simulink model "Kite"  (R2017b)
settings: Solver=VariableStepAuto  StartTime=0.0  StopTime=60  RelTol=1e-3  EnableMultiTasking=on
values from neighbouring files (symbols this model uses):
  A = 0.28    [init.m]    (also in main.m)
  beta0 = beta_star+betinho*pi/180    (= 0.436332312999)    [init.m]    (also in main.m)
  beta_star = 40*pi/180    (= 0.698131700798)    [init.m]    (also in main.m)
  beta_total = [y1 y2 y3 y4]    [init.m]    (also in main.m)
  dbeta0 = 0*pi/180    (= 0)    [init.m]    (also in main.m)
  delta_phi = 20*pi/180    (= 0.349065850399)    [init.m]    (also in main.m)
  dphi0 = -0.1*pi/180    (= -0.00174532925199)    [init.m]    (also in main.m)
  dr0 = 0    [init.m]    (also in main.m)
  g = 9.8    [init.m]    (also in main.m)
  imax = size    [init.m]    (also in main.m)
  L0 = L_0*pi/180    [init.m]    (also in main.m)
  m = 0.7    [init.m]    (also in main.m)
  phi0 = phi_star+phizinho*pi/180    (= 0.523598775598)    [init.m]    (also in main.m)
  phi_total = [x1 x2 x3 x4]    [init.m]    (also in main.m)
  r0 = rmin    (= 50)    [init.m]    (also in main.m)
  rmax = 275    [init.m]    (also in main.m = 250)
  rmin = 50    [init.m]    (also in main.m)
  Ro = 1.2    [init.m]    (also in main.m)
  vw = 10    [init.m]    (also in main.m)
settings Model: Creator=Gonçalo  LastModifiedBy=Conrado
settings SolverCC: MaxConsecutiveMinStep=10
settings OptimizationCC: LifeSpan=inf
settings DebuggingCC: SFUnexpectedBacktrackingDiag=warning  SFNoUnconditionalDefaultTransitionDiag=warning  SFExecutionAtInitializationDiag=none
settings CodeAppCC: StateflowObjectComments=on
settings GRTTargetCC: TargetLangStandard=C89/C90 (ANSI)
settings ConfigComp: CovMetricSettings=dw  CovSaveCumulativeToWorkspaceVar=on  CovSaveSingleToWorkspaceVar=on  CovExternalEMLEnable=off

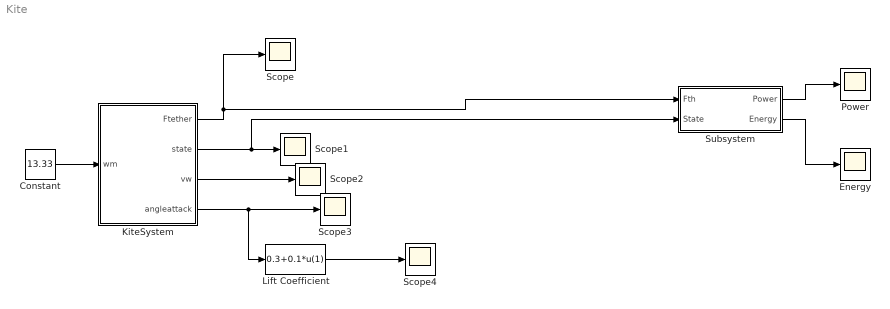
== system Kite ==
  Constant : Constant  Value=13.33
  "Energy " : Scope
  KiteSystem : Subsystem
  Lift Coefficient : Fcn  Expr=0.3+0.1*u(1)
  Power : Scope
  Scope{,1..4} (5 alike) : Scope
  Subsystem : Subsystem
  wires:
  Constant/1 -> KiteSystem/1(wm)
  KiteSystem/3("vw ") -> Scope2/1
  KiteSystem/4(angleattack) -> Lift Coefficient/1, Scope3/1
  Lift Coefficient/1 -> Scope4/1
  Subsystem/2("Energy ") -> "Energy "/1
  KiteSystem/2(state) -> Subsystem/2(State), Scope1/1
  Subsystem/1("Power ") -> Power/1
  KiteSystem/1(Ftether) -> Subsystem/1("Fth "), Scope/1

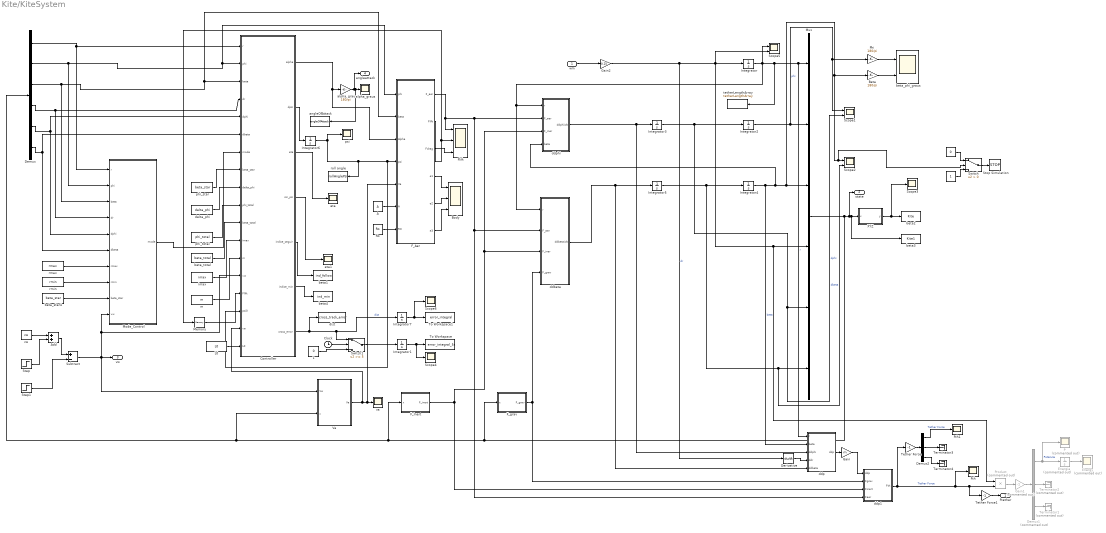
== system Kite/KiteSystem ==
  wm : Inport
  " " : Constant  Value=0
  " " : Constant
  " 1" : Constant  Value=0
  A : Constant  Value=A
  Add : Sum
  Beta : Gain  Gain=180/pi
  Body : Scope  NumInputPorts=3
  Clock : Clock
  Controller : MATLAB Function  TreatAsAtomicUnit=on
  Demux : Demux  Outputs=6
  Demux1 : Demux  Commented=on  Outputs=3
  Demux2 : Demux  Outputs=3
  Derivative : Derivative
  Energia : Integrator  Commented=on
  Energy : Scope  Commented=on
  F_Aer : Subsystem
  F_Inert : Subsystem
  F_grav : Subsystem
  Flift : Scope  NumInputPorts=3
  Fth : Scope
  Fth1 : Scope
  Gain : Gain  Gain=m
  Gain1 : Gain  Commented=on  Gain=-1
  Gain2 : Gain  Gain=0.25
  Integrator : Integrator  InitialCondition=r0
  Integrator1 : Integrator
  Integrator2 : Integrator  InitialCondition=phi0
  Integrator3 : Integrator  InitialCondition=dphi0
  Integrator4 : Integrator  InitialCondition=beta0
  Integrator5 : Integrator  InitialCondition=dbeta0
  Integrator6 : Integrator  InitialCondition=dr0
  Integrator7 : Integrator
  L0 : Constant  Value=L0
  Memory : Memory  InitialCondition=300
  Mode_Control : MATLAB Function  TreatAsAtomicUnit=on
  Mux : Mux  Inputs=6
  P : Scope  Commented=on
  Phi : Gain  Gain=180/pi
  Product : Product  Commented=on
  Ro : Constant  Value=Ro
  Scope1 : Scope  NumInputPorts=2
  Scope2 : Scope  NumInputPorts=2
  Scope3 : Scope
  Scope4 : Scope
  Scope5 : Scope  NumInputPorts=2
  Scope6 : Scope
  Step : Step  Time=25  After=0  SampleTime=0
  Step1 : Step  Time=27  After=0  SampleTime=0
  Stop Simulation : Stop
  Subtract : Sum  Inputs=+-
  Switch : Switch  Criteria=u2 > Threshold
  Switch1 : Switch  Threshold=5
  Terminator1 : Terminator  Commented=on
  Terminator2 : Terminator  Commented=on
  Terminator3 : Terminator
  Terminator4 : Terminator
  Tether Force : Gain  Gain=-1
  Tether Force1 : Gain  Gain=-1
  To Workspace : ToWorkspace  VariableName=error_integral_5s  SampleTime=-1
      settings: Save2DSignal=2-D array (concatenate along first dimension)
  To Workspace1 : ToWorkspace  VariableName=error_integral  SampleTime=-1
      settings: Save2DSignal=2-D array (concatenate along first dimension)
  Va : Subsystem
  XYZ : MATLAB Function  TreatAsAtomicUnit=on
  alpha_grau : Gain  Gain=180/pi
  alpha_graus : Scope
  angleOfAttack : ToWorkspace  VariableName=angleOfAttack  SampleTime=-1
      settings: Save2DSignal=2-D array (concatenate along first dimension)
  beta1 : ToWorkspace  VariableName=ind_follow  SampleTime=-1
      settings: Save2DSignal=2-D array (concatenate along first dimension)
  beta2 : ToWorkspace  VariableName=Kite  SampleTime=-1
      settings: Save2DSignal=2-D array (concatenate along first dimension)
  beta3 : ToWorkspace  VariableName=Kite1  SampleTime=-1
      settings: Save2DSignal=2-D array (concatenate along first dimension)
  beta4 : ToWorkspace  VariableName=ind_min  SampleTime=-1
      settings: Save2DSignal=2-D array (concatenate along first dimension)
  "beta_phi_graus " : Scope  NumInputPorts=2
  beta_star4 : Constant  Value=beta_star
  beta_total : Constant  Value=beta_total
  ddbeta : Subsystem
  ddp : Subsystem
  ddp1 : Subsystem
  ddphi : Subsystem
  delta_phi : Constant  Value=delta_phi
  dist : ToWorkspace  VariableName=cross_track_error  SampleTime=-1
      settings: Save2DSignal=2-D array (concatenate along first dimension)
  eta : Scope
  eta1 : Scope
  imax : Constant  Value=imax
  m : Constant  Value=m
  phi_star : Constant  Value=beta_star
  phi_total : Constant  Value=phi_total
  psi : Scope
  "rmax " : Constant  Value=rmax
  "rmin " : Constant  Value=rmin
  roll angle : ToWorkspace  VariableName=rollAnglePsi  SampleTime=-1
      settings: Save2DSignal=2-D array (concatenate along first dimension)
  tetherLengthArray : ToWorkspace  VariableName=tetherLengthArray  SampleTime=-1
      settings: Save2DSignal=2-D array (concatenate along first dimension)
  va : Scope
  vw : Constant  Value=vw
  Ftether : Outport
  state : Outport  Port=2
  "vw " : Outport  Port=3
  angleattack : Outport  Port=4
  wires:
  Integrator2/1 -> Scope1/1, Phi/1, Mux/2  "phi"
  Mode_Control/1(mode) -> Controller/7(mode)
  Integrator/1 -> Scope5/1, tetherLengthArray/1, ddp/1("r "), Mux/1, ddbeta/1(r), ddphi/1(r)  "r"
  beta_total/1 -> Controller/11(beta_total)
  imax/1 -> Controller/12(imax)
  Phi/1 -> "beta_phi_graus "/1
  Demux/1 -> Mode_Control/1(r), Controller/1(r)
  phi_star/1 -> Controller/8(beta_star)
  Subtract/1 -> "vw "/1, Controller/14(vw), Mode_Control/10(vw), Va/1("Vw ")
  Beta/1 -> "beta_phi_graus "/2
  Product/1 -> Gain1/1
  Demux/4 -> Mode_Control/4(dr), Controller/4(dr)
  phi_total/1 -> Controller/10(phi_total)
  Demux/2 -> Mode_Control/2(phi), Controller/2(phi), F_Aer/1("phi ")
  Demux1/3 -> Terminator1/1
  XYZ/1(y) -> Scope3/1, beta2/1
  A/1 -> F_Aer/6(A)
  Gain2/1 -> Derivative/1, Scope5/2, Product/1, Mux/4, Integrator/1  "dr"
  Mux/1 -> F_Inert/1("x "), Va/2(x), Demux/1, F_grav/1("x "), state/1, beta3/1, XYZ/1(x)
  Controller/2(dpsi) -> Integrator6/1
  ddp/1("ddp ") -> Gain/1
  ddbeta/1("ddbeta/dt ") -> Integrator5/1, ddp/5(ddbeta)
  Demux/3 -> Mode_Control/3(beta), F_Aer/2(beta), Controller/3(beta)
  F_Inert/1("F_inert ") -> ddphi/3(F_iner), ddbeta/3(F_iner), ddp1/3(Finert)
  Integrator4/1 -> ddp/2(beta), ddphi/4(beta), Switch/2, Scope2/1, Beta/1, Mux/3  "beta"
  ddphi/1("ddphi/dt ") -> ddp/3("ddphi "), Integrator3/1
  Integrator3/1 -> Integrator2/1, Scope1/2, Mux/5  "dphi"
  Integrator5/1 -> Integrator4/1, Scope2/2, Mux/6  "dbeta"
  Demux/5 -> Mode_Control/5(dphi), Controller/5(dphi)
  F_Aer/2(Flift) -> Flift/2, Memory/1
  Demux2/3 -> Terminator4/1
  F_Aer/3(Fdrag) -> Flift/3
  delta_phi/1 -> Controller/9(delta_phi)
  F_Aer/1("F_aer ") -> ddp1/4("Faer "), ddbeta/2(F_aer), ddphi/2(F_aer), Flift/1
  Demux/6 -> Mode_Control/6(dbeta), Controller/6(dbeta)
  m/1 -> Controller/13(m)
  Step/1 -> Add/2
  Ro/1 -> F_Aer/7(R0)
  vw/1 -> Add/1
  Controller/1(alpha) -> alpha_grau/1, F_Aer/3(Alpha)
  Gain1/1 -> Demux1/1
  Demux1/2 -> Terminator2/1
  "rmin "/1 -> Mode_Control/8(rmin)
  Demux1/1 -> P/1, Energia/1  "Potência"
  F_Aer/6(e3) -> Body/3
  Tether Force/1 -> Demux2/1
  Integrator6/1 -> roll angle/1, Controller/16(psi0), F_Aer/4(psi), psi/1
  "rmax "/1 -> Mode_Control/7(rmax)
  F_Aer/4(e1) -> Body/1
  Va/1("Va ") -> Controller/17(va), va/1, F_Aer/5(Va)
  F_Aer/5(e2) -> Body/2
  Add/1 -> Subtract/1
  Memory/1 -> Controller/15(Flift)
  Gain/1 -> ddp1/1(ddp)
  F_grav/1("F_grav ") -> ddbeta/4(F_grav), ddp1/2(Fgrav)
  " "/1 -> Switch/1
  beta_star4/1 -> Mode_Control/9(beta_star)
  Demux2/1 -> Fth1/1  "Tether Force"
  Energia/1 -> Energy/1
  " "/1 -> Switch/3
  Demux2/2 -> Terminator3/1
  Step1/1 -> Subtract/2
  Switch/1 -> Stop Simulation/1
  wm/1 -> Gain2/1
  Derivative/1 -> ddp/4(ddr)
  alpha_grau/1 -> angleattack/1, angleOfAttack/1, alpha_graus/1
  ddp1/1("Fth ") -> Tether Force1/1, Product/2, Fth/1, Tether Force/1  "Tether Force"
  Tether Force1/1 -> Ftether/1
  Controller/4(sin_psi) -> eta1/1
  Controller/3(eta) -> eta/1
  Controller/5(indice_seguir) -> beta1/1
  Controller/6(indice_min) -> beta4/1
  L0/1 -> Controller/18(L0)
  Controller/7(cross_error) -> Switch1/1, Integrator7/1, dist/1  "dist"
  Integrator1/1 -> To Workspace/1, Scope4/1
  Switch1/1 -> Integrator1/1
  Clock/1 -> Switch1/2
  Integrator7/1 -> Scope6/1, To Workspace1/1
  " 1"/1 -> Switch1/3

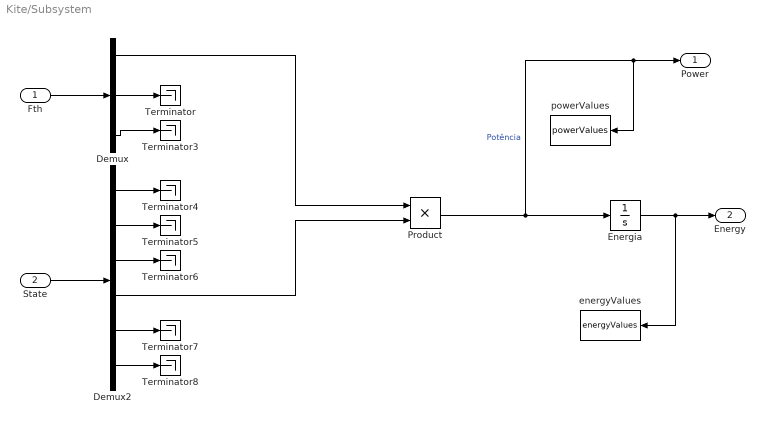
== system Kite/Subsystem ==
  "Fth " : Inport
  State : Inport  Port=2
  Demux : Demux  Outputs=3
  Demux2 : Demux  Outputs=6
  Energia : Integrator
  Product : Product
  Terminator{,3..8} (7 alike) : Terminator
  energyValues : ToWorkspace  VariableName=energyValues  SampleTime=-1
      settings: Save2DSignal=2-D array (concatenate along first dimension)
  powerValues : ToWorkspace  VariableName=powerValues  SampleTime=-1
      settings: Save2DSignal=2-D array (concatenate along first dimension)
  "Power " : Outport
  "Energy " : Outport  Port=2
  wires:
  Product/1 -> Energia/1, powerValues/1, "Power "/1  "Potência"
  Energia/1 -> energyValues/1, "Energy "/1
  "Fth "/1 -> Demux/1
  State/1 -> Demux2/1
  Demux/2 -> Terminator/1
  Demux/3 -> Terminator3/1
  Demux2/1 -> Terminator4/1
  Demux2/2 -> Terminator5/1
  Demux2/3 -> Terminator6/1
  Demux2/5 -> Terminator7/1
  Demux2/6 -> Terminator8/1
  Demux2/4 -> Product/2
  Demux/1 -> Product/1

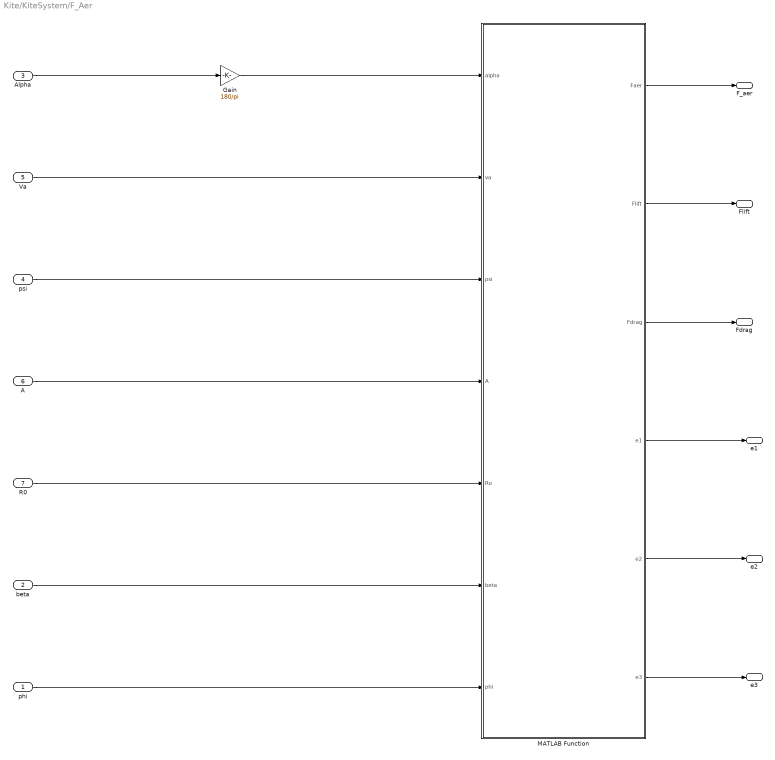
== system Kite/KiteSystem/F_Aer ==
  "phi " : Inport
  beta : Inport  Port=2
  Alpha : Inport  Port=3
  psi : Inport  Port=4
  Va : Inport  Port=5
  A : Inport  Port=6
  R0 : Inport  Port=7
  Gain : Gain  Gain=180/pi
  MATLAB Function : MATLAB Function  TreatAsAtomicUnit=on
  "F_aer " : Outport
  Flift : Outport  Port=2
  Fdrag : Outport  Port=3
  e1 : Outport  Port=4
  e2 : Outport  Port=5
  e3 : Outport  Port=6
  wires:
  Alpha/1 -> Gain/1
  Va/1 -> MATLAB Function/2(va)
  psi/1 -> MATLAB Function/3(psi)
  A/1 -> MATLAB Function/4(A)
  R0/1 -> MATLAB Function/5(Ro)
  MATLAB Function/1(Faer) -> "F_aer "/1
  beta/1 -> MATLAB Function/6(beta)
  "phi "/1 -> MATLAB Function/7(phi)
  Gain/1 -> MATLAB Function/1(alpha)
  MATLAB Function/2(Flift) -> Flift/1
  MATLAB Function/3(Fdrag) -> Fdrag/1
  MATLAB Function/4(e1) -> e1/1
  MATLAB Function/5(e2) -> e2/1
  MATLAB Function/6(e3) -> e3/1

== system Kite/KiteSystem/F_Inert ==
  "x " : Inport
  Add : Sum
  Fcent : Subsystem
  Fcor : Subsystem
  "F_inert " : Outport
  wires:
  Add/1 -> "F_inert "/1
  "x "/1 -> Fcent/1(x), Fcor/1(x)
  Fcent/1(Fcent) -> Add/1
  Fcor/1(Fcor) -> Add/2

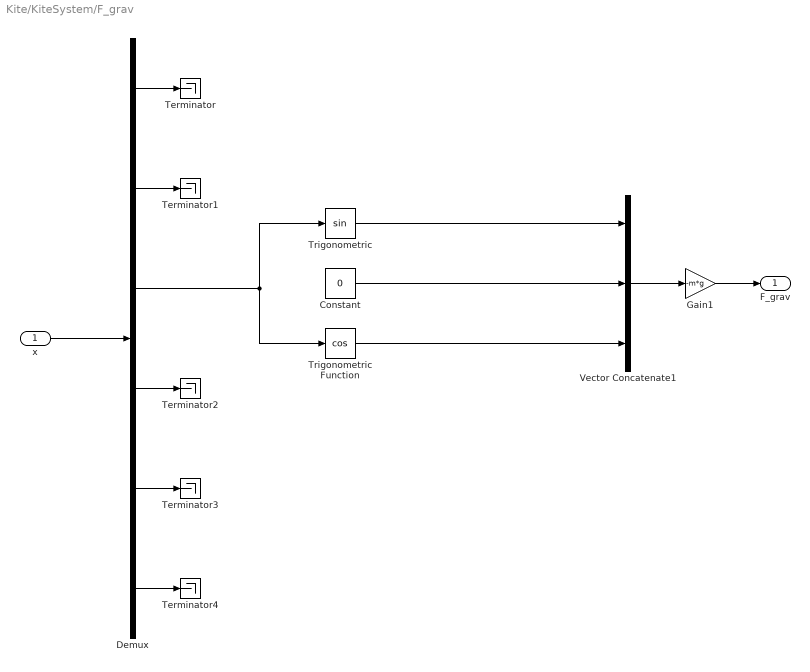
== system Kite/KiteSystem/F_grav ==
  "x " : Inport
  Constant : Constant  Value=0
  Demux : Demux  Outputs=6
  Gain1 : Gain  Gain=-m*g
  Terminator{,1..4} (5 alike) : Terminator
  Trigonometric : Trigonometry
  Trigonometric Function : Trigonometry  Operator=cos
  Vector Concatenate1 : Concatenate  NumInputs=3  Mode=Multidimensional array
  "F_grav " : Outport
  wires:
  Vector Concatenate1/1 -> Gain1/1
  Gain1/1 -> "F_grav "/1
  Trigonometric/1 -> Vector Concatenate1/1
  Demux/1 -> Terminator/1
  Demux/3 -> Trigonometric Function/1, Trigonometric/1
  Demux/4 -> Terminator2/1
  "x "/1 -> Demux/1
  Demux/2 -> Terminator1/1
  Demux/5 -> Terminator3/1
  Demux/6 -> Terminator4/1
  Trigonometric Function/1 -> Vector Concatenate1/3
  Constant/1 -> Vector Concatenate1/2

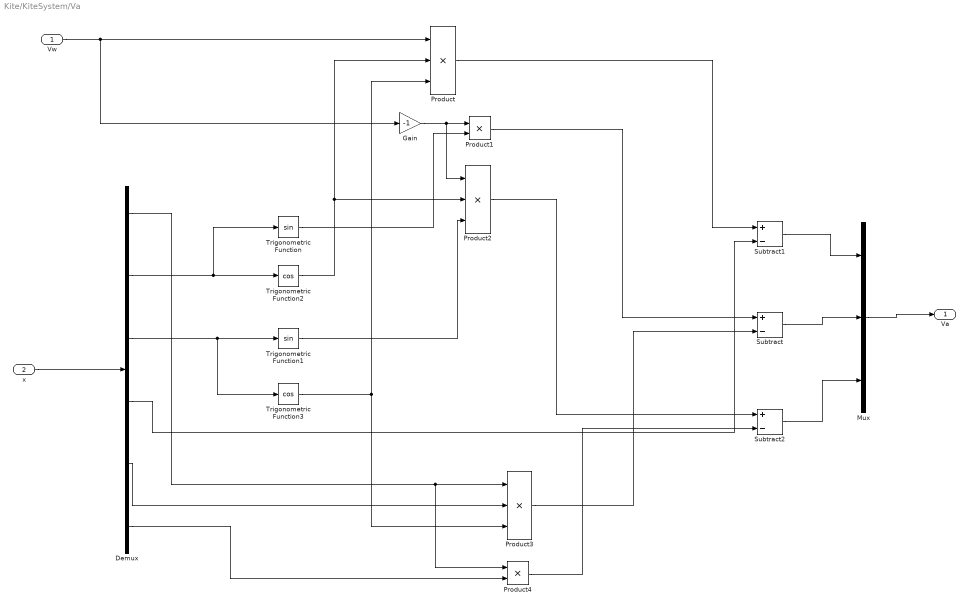
== system Kite/KiteSystem/Va ==
  "Vw " : Inport
  x : Inport  Port=2
  Demux : Demux  Outputs=6
  Gain : Gain  Gain=-1
  Mux : Mux  Inputs=3
  Product : Product  Inputs=3
  Product1 : Product
  Product2 : Product  Inputs=3
  Product3 : Product  Inputs=3
  Product4 : Product
  Subtract : Sum  Inputs=+-
  Subtract1 : Sum  Inputs=+-
  Subtract2 : Sum  Inputs=+-
  Trigonometric Function : Trigonometry
  Trigonometric Function1 : Trigonometry
  Trigonometric Function2 : Trigonometry  Operator=cos
  Trigonometric Function3 : Trigonometry  Operator=cos
  "Va " : Outport
  wires:
  x/1 -> Demux/1
  Demux/2 -> Trigonometric Function2/1, Trigonometric Function/1
  Demux/3 -> Trigonometric Function3/1, Trigonometric Function1/1
  "Vw "/1 -> Gain/1, Product/1
  Trigonometric Function2/1 -> Product2/2, Product/2
  Trigonometric Function3/1 -> Product3/3, Product/3
  Product1/1 -> Subtract/1
  Product/1 -> Subtract1/1
  Gain/1 -> Product2/1, Product1/1
  Product3/1 -> Subtract/2
  Demux/4 -> Subtract1/2
  Demux/1 -> Product3/1, Product4/1
  Product4/1 -> Subtract2/2
  Trigonometric Function/1 -> Product1/2
  Trigonometric Function1/1 -> Product2/3
  Demux/5 -> Product3/2
  Demux/6 -> Product4/2
  Product2/1 -> Subtract2/1
  Subtract1/1 -> Mux/1
  Mux/1 -> "Va "/1
  Subtract/1 -> Mux/2
  Subtract2/1 -> Mux/3

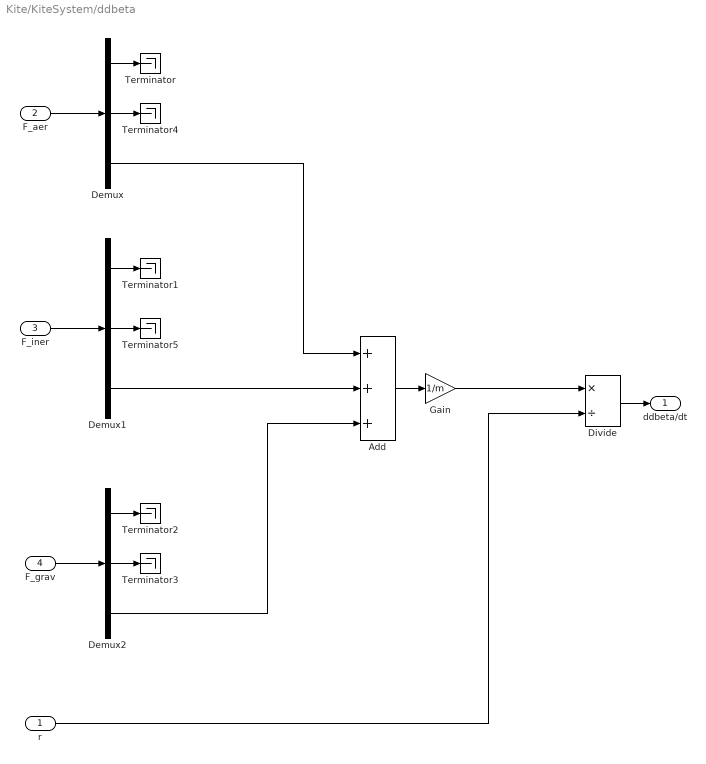
== system Kite/KiteSystem/ddbeta ==
  r : Inport
  F_aer : Inport  Port=2
  F_iner : Inport  Port=3
  F_grav : Inport  Port=4
  Add : Sum  Inputs=+++
  Demux : Demux  Outputs=3
  Demux1 : Demux  Outputs=3
  Demux2 : Demux  Outputs=3
  Divide : Product  Inputs=*/
  Gain : Gain  Gain=1/m
  Terminator{,1..5} (6 alike) : Terminator
  "ddbeta/dt " : Outport
  wires:
  Gain/1 -> Divide/1
  Add/1 -> Gain/1
  F_aer/1 -> Demux/1
  Demux/1 -> Terminator/1
  F_iner/1 -> Demux1/1
  Demux1/1 -> Terminator1/1
  Divide/1 -> "ddbeta/dt "/1
  r/1 -> Divide/2
  F_grav/1 -> Demux2/1
  Demux2/1 -> Terminator2/1
  Demux2/3 -> Add/3
  Demux2/2 -> Terminator3/1
  Demux/2 -> Terminator4/1
  Demux/3 -> Add/1
  Demux1/3 -> Add/2
  Demux1/2 -> Terminator5/1

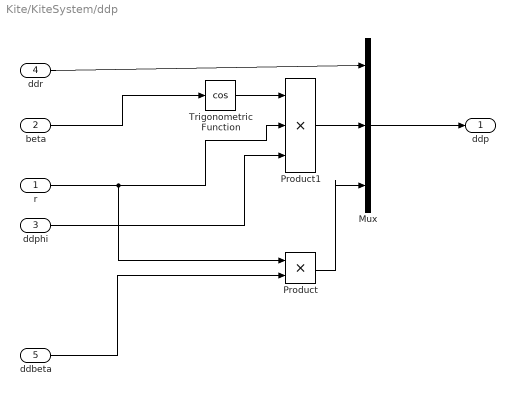
== system Kite/KiteSystem/ddp ==
  "r " : Inport
  beta : Inport  Port=2
  "ddphi " : Inport  Port=3
  ddr : Inport  Port=4
  ddbeta : Inport  Port=5
  Mux : Mux  Inputs=3
  Product : Product
  Product1 : Product  Inputs=3
  Trigonometric Function : Trigonometry  Operator=cos
  "ddp " : Outport
  wires:
  Mux/1 -> "ddp "/1
  ddr/1 -> Mux/1
  ddbeta/1 -> Product/2
  Product/1 -> Mux/3
  "r "/1 -> Product1/2, Product/1
  Product1/1 -> Mux/2
  Trigonometric Function/1 -> Product1/1
  beta/1 -> Trigonometric Function/1
  "ddphi "/1 -> Product1/3

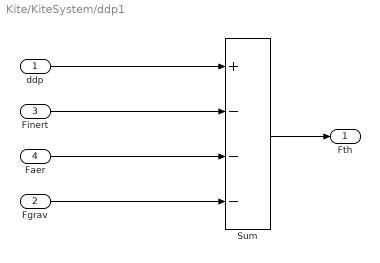
== system Kite/KiteSystem/ddp1 ==
  ddp : Inport
  Fgrav : Inport  Port=2
  Finert : Inport  Port=3
  "Faer " : Inport  Port=4
  Sum : Sum  Inputs=+---
  "Fth " : Outport
  wires:
  ddp/1 -> Sum/1
  Finert/1 -> Sum/2
  "Faer "/1 -> Sum/3
  Sum/1 -> "Fth "/1
  Fgrav/1 -> Sum/4

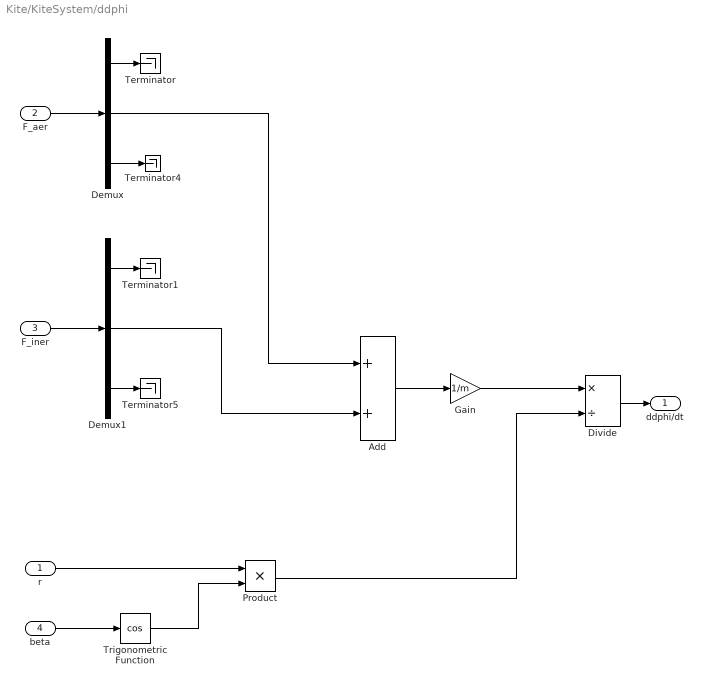
== system Kite/KiteSystem/ddphi ==
  r : Inport
  F_aer : Inport  Port=2
  F_iner : Inport  Port=3
  beta : Inport  Port=4
  Add : Sum
  Demux : Demux  Outputs=3
  Demux1 : Demux  Outputs=3
  Divide : Product  Inputs=*/
  Gain : Gain  Gain=1/m
  Product : Product
  Terminator{,1,4..5} (4 alike) : Terminator
  Trigonometric Function : Trigonometry  Operator=cos
  "ddphi/dt " : Outport
  wires:
  Gain/1 -> Divide/1
  Add/1 -> Gain/1
  F_aer/1 -> Demux/1
  Demux/1 -> Terminator/1
  F_iner/1 -> Demux1/1
  Demux1/1 -> Terminator1/1
  Divide/1 -> "ddphi/dt "/1
  Demux/3 -> Terminator4/1
  Demux1/3 -> Terminator5/1
  Demux/2 -> Add/1
  Demux1/2 -> Add/2
  beta/1 -> Trigonometric Function/1
  r/1 -> Product/1
  Trigonometric Function/1 -> Product/2
  Product/1 -> Divide/2

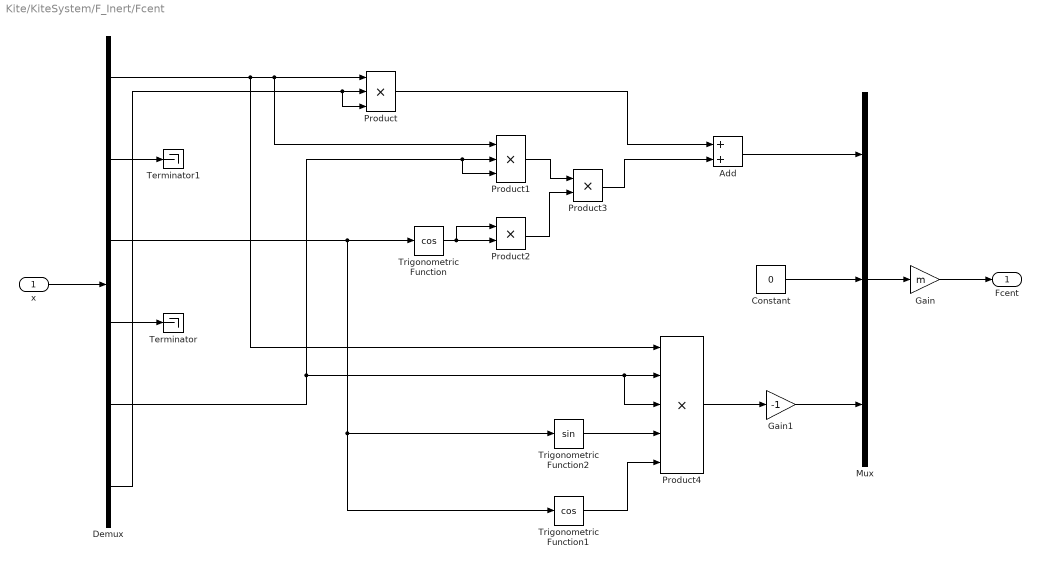
== system Kite/KiteSystem/F_Inert/Fcent ==
  x : Inport
  Add : Sum
  Constant : Constant  Value=0
  Demux : Demux  Outputs=6
  Gain : Gain  Gain=m
  Gain1 : Gain  Gain=-1
  Mux : Mux  Inputs=3
  Product : Product  Inputs=3
  Product1 : Product  Inputs=3
  Product2 : Product
  Product3 : Product
  Product4 : Product  Inputs=5
  Terminator : Terminator
  Terminator1 : Terminator
  Trigonometric Function : Trigonometry  Operator=cos
  Trigonometric Function1 : Trigonometry  Operator=cos
  Trigonometric Function2 : Trigonometry
  Fcent : Outport
  wires:
  x/1 -> Demux/1
  Gain/1 -> Fcent/1
  Mux/1 -> Gain/1
  Demux/1 -> Product4/1, Product1/1, Product/1
  Demux/3 -> Trigonometric Function1/1, Trigonometric Function2/1, Trigonometric Function/1
  Trigonometric Function/1 -> Product2/1, Product2/2
  Product1/1 -> Product3/1
  Product2/1 -> Product3/2
  Product3/1 -> Add/2
  Product/1 -> Add/1
  Add/1 -> Mux/1
  Constant/1 -> Mux/2
  Gain1/1 -> Mux/3
  Product4/1 -> Gain1/1
  Trigonometric Function2/1 -> Product4/4
  Trigonometric Function1/1 -> Product4/5
  Demux/4 -> Terminator/1
  Demux/5 -> Product4/3, Product4/2, Product1/3, Product1/2
  Demux/6 -> Product/3, Product/2
  Demux/2 -> Terminator1/1

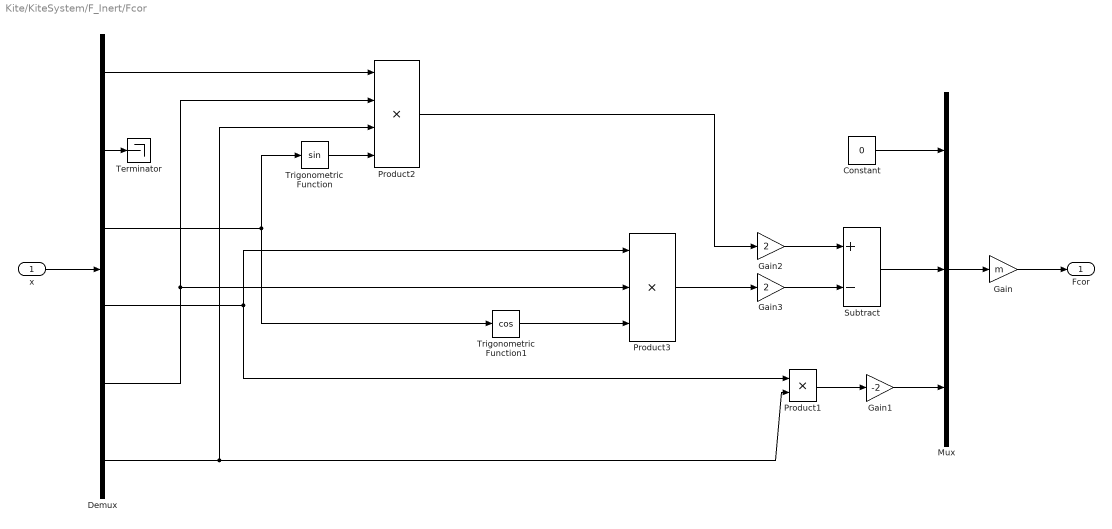
== system Kite/KiteSystem/F_Inert/Fcor ==
  x : Inport
  Constant : Constant  Value=0
  Demux : Demux  Outputs=6
  Gain : Gain  Gain=m
  Gain1 : Gain  Gain=-2
  Gain2 : Gain  Gain=2
  Gain3 : Gain  Gain=2
  Mux : Mux  Inputs=3
  Product1 : Product
  Product2 : Product  Inputs=4
  Product3 : Product  Inputs=3
  Subtract : Sum  Inputs=+-
  Terminator : Terminator
  Trigonometric Function : Trigonometry
  Trigonometric Function1 : Trigonometry  Operator=cos
  Fcor : Outport
  wires:
  x/1 -> Demux/1
  Gain/1 -> Fcor/1
  Mux/1 -> Gain/1
  Constant/1 -> Mux/1
  Gain1/1 -> Mux/3
  Product1/1 -> Gain1/1
  Demux/4 -> Product1/1, Product3/1
  Demux/1 -> Product2/1
  Demux/5 -> Product2/2, Product3/2
  Demux/6 -> Product2/3, Product1/2
  Product2/1 -> Gain2/1
  Trigonometric Function/1 -> Product2/4
  Demux/3 -> Trigonometric Function/1, Trigonometric Function1/1
  Gain2/1 -> Subtract/1
  Subtract/1 -> Mux/2
  Product3/1 -> Gain3/1
  Gain3/1 -> Subtract/2
  Demux/2 -> Terminator/1
  Trigonometric Function1/1 -> Product3/3

== matlab function Kite/KiteSystem/F_Aer/MATLAB Function ==
  data: alpha input; Faer output; va input; psi input; A input; Ro input; beta input; phi input; Flift output; Fdrag output; e1 output; e2 output; e3 output
function [Faer, Flift, Fdrag, e1, e2, e3]   = fcn(alpha, va,psi, A, Ro, beta, phi)
%#codegen

% if alpha > 12
%     Cl=9.9-0.7*alpha;
% else
   Cl=0.3+0.1*alpha;
% end
if alpha>=0
Cd= 0.012+0.01*alpha;
else
    Cd=0.012-0.01*alpha;
end
Faer = zeros(3,1);
Flift = zeros(3,1);
Fdrag= zeros(3,1);

% RGL=[cos(beta)*cos(phi) cos(beta)*sin(phi)  sin(beta);
%     -sin(phi)           cos(phi)            0;
%     -sin(beta)*cos(phi) -sin(beta)*sin(phi) cos(beta)];
% 
% er=RGL*[0;0;1];
er=[1;0;0];
e1=[0;0;0];
e2=[0;0;0];
e3=[0;0;0];

e1 = -va/norm(va);

aux=cross(er,e1);

f2=aux/norm(aux);

e2=f2*cos(psi)+cross(e1,f2)*sin(psi)+e1*(dot(e1,f2))*(1-cos(psi));

e3=cross(e1,e2);

Flift= 0.5*Ro*A*norm(va)^2*Cl*e3;
Fdrag= 0.5*Ro*A*norm(va)^2*Cd*e1;
Faer=Flift-Fdrag;

%Faer = 0.5*Ro*A*norm(va)^2*Cl*e3-0.5*Ro*A*norm(va)^2*Cd*e1;

end

== matlab function Kite/KiteSystem/Mode_Control ==
  data: r input; phi input; beta input; dr input; dphi input; dbeta input; rmax input; rmin input; beta_star input; mode output; vw input
function mode = fcn(r, phi, beta, dr, dphi, dbeta, rmax, rmin, beta_star, vw)
% 2 modos apenas: 
% Modo 1: Reel-out
% Modo 2: Ir para Beta Star
% Modo 3: Fast Reel-in

%

% if vw>=25
%     mode=2;
%     AA=2;
% elseif r>=rmax+5 && dr>0 %&& dphi>=0
%     mode=2;
%     AA=2;
% elseif r>rmax && dr>0 && phi<0 && dphi>0
%     mode = 5;
%     AA=5;
% elseif dr<=0 && r>rmin
%     mode=3;
%     AA=3;
% elseif dr<0 && r<rmin
%     mode=4;
%     AA=4;
% else
    mode=1;
% end



% if dr >= 0
%     if r < rmax
%         
%         mode = 1;   % Fase produção
%         AA=1;
%     else % r<= rmax
%         mode = 2;
%         AA=2;
%     end
%     
%     
%     
% else % dr < 0
%     
%     if r > rmin
%             mode = 2;   % Chega a rmax, passa a Reel-in
%             AA=3;
%         else
%             mode = 1;   % Chega a rmin, passa a fase produção
%             AA=4;
%               
%     end
% end 


   
end

== matlab function Kite/KiteSystem/Controller ==
  data: r input; phi input; beta input; dr input; dphi input; dbeta input; mode input; beta_star input; delta_phi input; phi_total input; beta_total input; imax input; m input; vw input; alpha output; dpsi output size=1; Flift input; psi0 input; va input; eta output; sin_psi output; indice_seguir output; indice_min output; L0 input; cross_error output
function [alpha, dpsi, eta, sin_psi, indice_seguir, indice_min, cross_error]  = fcn(r, phi, beta, dr, dphi, dbeta, mode, beta_star, delta_phi,phi_total, beta_total, imax, m, vw, Flift, psi0, va, L0)
% phi
v_producao = vw/3;%vw/5%vw/8
Ro=1.225;A=0.28;g=9.81;
size=length(phi_total);
% r_total=(r+v_producao)*ones(1,size);
% r_total=(r+0.5)*ones(1,size);
r_total=(r+dr)*ones(1,size);%(r+v_producao)*ones(1,size);
% r_total=r*ones(1,size);%(r+v_producao)*ones(1,size);
phi_total=phi_total';
beta_total=beta_total';
% Trajetorias
% Traj_L=[r_total;
%         phi_total;
%         beta_total];
Traj_L=[ phi_total;
        beta_total];
% Traj_G=[r_total.*cos(beta_total).*cos(phi_total);
%         r_total.*cos(beta_total).*sin(phi_total);
%         r_total.*sin(beta_total)];
% Coordenadas Esféricas
% pL=[r;
%     phi;
%     beta];
%
% dpL=[dr;
%      r*dphi*cos(beta);
%      r*dbeta];
 pL=[phi;
    beta];
dpL=[0;%dr;
    r*dphi*cos(beta);
     r*dbeta];
% Cordenadas Cartesianas
% pG=[r.*cos(beta).*cos(phi);
%     r.*cos(beta).*sin(phi);
%     r.*sin(beta)];
% Descobrir ponto mais próximo
% dist=sqrt((Traj_L(1,:)-pL(1)).^2+(Traj_L(2,:)-pL(2)).^2+(Traj_L(3,:)-pL(3)).^2);
% dist=sqrt((Traj_L(2,:)-pL(2)).^2+(Traj_L(3,:)-pL(3)).^2);
dist=sqrt((phi_total-phi).^2+(beta_total-beta).^2);

[~, indice_min]=min(dist);

%L0=5*pi/180;

%Cross Track Error
cross_error = sqrt((phi_total(indice_min)-phi).^2+(beta_total(indice_min)-beta).^2);

dist_QR=sqrt((phi_total-phi_total(indice_min)).^2+(beta_total-beta_total(indice_min)).^2)-L0;

for k=1:length(dist_QR)
    if dist_QR(k)<0
        dist_QR(k)=1000;
    end
end
[~, indice_seg1]=min(dist_QR);
aux1=dist_QR(indice_seg1);
dist_QR(indice_seg1)=1000;
[~,indice_seg2]=min(dist_QR);
aux2=dist_QR(indice_seg2);
coiso=[aux1 aux2];
if indice_seg1>imax
    indice_seg1=indice_seg1-imax;
end
if indice_seg2>imax
    indice_seg2=indice_seg2-imax;
end
% indice_seguir=indice_min+10;%+4
%
% if indice_seguir>imax
%     indice_seguir=indice_seguir-imax;
% end
L1_a=[0;%Traj_L(1, indice_min)-pL(1);
      phi_total(indice_seg1)-phi;%Traj_L(2, indice_min)-pL(2);
      beta_total(indice_seg1)-beta];%Traj_L(3, indice_min)-pL(3)];
L1_b=[0;%Traj_L(1, indice_min2)-pL(1);
      phi_total(indice_seg2)-phi;%Traj_L(2, indice_min2)-pL(2);
      beta_total(indice_seg2)-beta];%Traj_L(3, indice_min2)-pL(3)];
if dot(dpL,L1_a)>dot(dpL,L1_b)
    L1_L=L1_a;
%     L1_G=L1_Ga;
    indice_seguir=indice_seg1;
else
    L1_L=L1_b;
%     L1_G=L1_Gb;
    indice_seguir=indice_seg2;
end
L1_L=[0;%r_total(indice_seguir)-r;
      phi_total(indice_seguir)-phi;
      beta_total(indice_seguir)-beta];
  n=-[1;0;0];
  
%   QR=[dpL(1)-r; dpL(2)-phi; dpL(3)-beta ];
% QS=L1_L;%[r_total(indice_seguir)-r; L1_L(2)-phi; L1_L(3)-beta];
% % 
% n=[QR(2)*QS(3)-QR(3)*QS(2); QR(3)*QS(1)-QR(1)*QS(3); QR(1)*QS(2)-QR(2)*QS(1)];
% n=-n/norm(n);
aux1=cross(dpL,L1_L);%=a*b*sin(eta)*n
% aux1=cross(L1_L,dpL);
aux2=aux1/norm(aux1);
aux2=aux1/(norm(dpL)*norm(L1_L));
aux3=dot(dpL,L1_L);
aux4=aux3/norm(aux3);
aux4=aux3/(norm(dpL)*norm(L1_L));
eta=atan2(dot(aux2,n),aux4);
% if eta>pi/2
%     eta=pi/2;
% elseif eta<-pi/2
%     eta=-pi/2;
% end
% % 
% % L1_G=[Traj_G(1, indice_seguir)-pG(1);  
% %       Traj_G(2, indice_seguir)-pG(2);  
% %       Traj_G(3, indice_seguir)-pG(3)];  
% 
% % n=[1;0;0];
% QR=[dpL(1)-r; dpL(2)-phi; dpL(3)-beta ];
% QS=[L1_L(1)-r; L1_L(2)-phi; L1_L(3)-beta];
% 
% n=[QR(2)*QS(3)-QR(3)*QS(2); QR(3)*QS(1)-QR(1)*QS(3); QR(1)*QS(2)-QR(2)*QS(1)];
% 
% sin_eta=cross(dpL,L1_L)./(norm(dpL)*norm(L1_L)*n);
% % cos_eta=dot(dpL,L1_L)/(norm(dpL)*norm(L1_L));
% %gamma=atan2(dpL(2)*L1_L(3)-dpL(3)*L1_L(2),dpL(2)*dpL(3)+L1_L(2)*L1_L(3));
% if sin_eta(1)>1
%     sin_eta(1)=1;
% elseif sin_eta(1)<-1
%     sin_eta(1)=-1;
% end
% eta=asin(sin_eta(1));%*2;%*360/pi;
% % if eta>pi/3
% %     eta=pi/3;
% % elseif eta<-pi/3
% %     eta=-pi/3;
% % end
% % eta=acos(cos_eta);
% % gamma=asin(sin_gamma(1));

% 
% norma_dp=norm(dpL);
% seno_gamma=sin(gamma);
% norma_Flift=norm(Flift(2:3));
% normaL1=norm(L1_G);

sin_psi=2*m*(norm(dpL)^2*sin(eta))/(norm(Flift)*(norm(L1_L)));%question this

if sin_psi < -sqrt(3)/2
    sin_psi=-sqrt(3)/2;
elseif sin_psi > sqrt(3)/2
    sin_psi=sqrt(3)/2;
end

% if mode==1
psi=asin(sin_psi);
dpsi=-10*(1/(m*(1.385/2)^2))*(psi0-psi); %based on a simple calculation of inertia K/I (K=10)
alpha=10*pi/180;
% at=0.05*(v_producao-dr);

% elseif mode==2
% 
% % dpsi=1*(0-pL(2));
% % alpha=5*pi/180;
% % at=0.5*(-0.3-dr);
% 
% 
% phi_ref=0;
% b_fl=norm(Flift)/(m*r*cos(beta));
% f_fl=(-2*m*dr*dphi*cos(beta)+2*m*r*dphi*dbeta*sin(beta))/(m*r*cos(beta));
% KP_fl=-1;
% KD_fl=-2;
% v_fl=KP_fl*(phi-phi_ref)+KD_fl*dphi;
% sin_psi=(v_fl-f_fl)/b_fl;
% if sin_psi < -1
%     sin_psi=-1;
% elseif sin_psi > 1
%     sin_psi=1;
% end
% 
% psi=asin(sin_psi);
% 
% dpsi=-10*(1/(m*(1.385/2)^2))*(psi0-psi);
% 
% 
% 
% beta_ref=80*pi/180;
% aux1=0.5*Ro*A*norm(va)^2;
% aux2=1/(m*r);
% e1=-va/(norm(va));
% e3=[0 0 1];
% head=dot(e1,e3);
% 
% b_alp=aux1*aux2*(-0.7*sin(psi0)*sin(beta)*sin(acos(head))-0.01*cos(beta)*head);
% f_alp=aux2*(-m*g*cos(beta)+2*m*dr*dbeta+m*r*dphi^2*cos(beta)*sin(beta)-aux1*(9.9*sin(psi0)*sin(acos(head))*sin(beta)-0.012*cos(beta)*head));
% 
% KP_alp=-9;
% KD_alp=-6;
% v_alp=KP_alp*(beta-beta_ref)+KD_alp*dbeta;
% alpha=(pi/180)*(v_alp-f_alp)/b_alp;
% 
% 
% 
% 
% % at=0.5*(-0.1-dr);
% 
% elseif mode==5
%     phi_ref=0;
% b_fl=norm(Flift)/(m*r*cos(beta));
% f_fl=(-2*m*dr*dphi*cos(beta)+2*m*r*dphi*dbeta*sin(beta))/(m*r*cos(beta));
% KP_fl=-1;
% KD_fl=-2;
% v_fl=KP_fl*(phi-phi_ref)+KD_fl*dphi;
% sin_psi=(v_fl-f_fl)/b_fl;
% if sin_psi < -1
%     sin_psi=-1;
% elseif sin_psi > 1
%     sin_psi=1;
% end
% 
% psi=asin(sin_psi);
% % psi=1*(0-pL(2));
% dpsi=-10*(1/(m*(1.385/2)^2))*(psi0-psi);
% % alpha=5*pi/180;
% 
% 
% beta_ref=80*pi/180;
% aux1=0.5*Ro*A*norm(va)^2;
% aux2=1/(m*r);
% e1=-va/(norm(va));
% e3=[0 0 1];
% head=dot(e1,e3);
% 
% b_alp=aux1*aux2*(-0.7*sin(psi0)*sin(beta)*sin(acos(head))-0.01*cos(beta)*head);
% f_alp=aux2*(-m*g*cos(beta)+2*m*dr*dbeta+m*r*dphi^2*cos(beta)*sin(beta)-aux1*(9.9*sin(psi0)*sin(acos(head))*sin(beta)-0.012*cos(beta)*head));
% 
% KP_alp=-1;
% KD_alp=-2;
% v_alp=KP_alp*(beta-beta_ref)+KD_alp*dbeta;
% alpha=(pi/180)*(v_alp-f_alp)/b_alp;
% 
% % at=0.5*(0-dr);
% 
% elseif mode==4
%     phi_ref=0*pi/180;
% b_fl=norm(Flift)/(m*r*cos(beta));
% f_fl=(-2*m*dr*dphi*cos(beta)+2*m*r*dphi*dbeta*sin(beta))/(m*r*cos(beta));
% KP_fl=-1;
% KD_fl=-2;
% v_fl=KP_fl*(phi-phi_ref)+KD_fl*dphi;
% sin_psi=(v_fl-f_fl)/b_fl;
% if sin_psi < -1
%     sin_psi=-1;
% elseif sin_psi > 1
%     sin_psi=1;
% end
% 
% psi=asin(sin_psi);
% % psi=1*(0-pL(2));
% dpsi=-10*(1/(m*(1.385/2)^2))*(psi0-psi);
% 
% 
% Ro=1.225;A=0.28;g=9.81;
% beta_ref=40*pi/180;
% aux1=0.5*Ro*A*norm(va)^2;
% aux2=1/(m*r);
% e1=-va/(norm(va));
% e3=[0 0 1];
% head=dot(e1,e3);
% % aux3=0.1*sin(beta_ref-beta)-0.01*cos(beta_ref-beta);
% % aux4=-0.3*sin(beta_ref-beta)+0.012*cos(beta_ref-beta);
% % 
% % alpha=(pi/180)*(((m*g*cos(beta_ref-beta))/aux1)+aux4)/aux3;
% 
% b_alp=aux1*aux2*(0.1*sin(psi0)*sin(beta)*sin(acos(head))-0.01*cos(beta)*head);
% f_alp=aux2*(-m*g*cos(beta)+2*m*dr*dbeta+m*r*dphi^2*cos(beta)*sin(beta)-aux1*(0.3*sin(psi0)*sin(acos(head))*sin(beta)-0.012*cos(beta)*head));
% 
% KP_alp=-9;
% KD_alp=-6;
% v_alp=KP_alp*(beta-beta_ref)+KD_alp*dbeta;
% alpha=(pi/180)*(v_alp-f_alp)/b_alp;
% 
% % at=0.1*(0.1-dr);
% else
% 
%     
% phi_ref=0;
% b_fl=norm(Flift)/(m*r*cos(beta));
% f_fl=(-2*m*dr*dphi*cos(beta)+2*m*r*dphi*dbeta*sin(beta))/(m*r*cos(beta));
% KP_fl=-9;
% KD_fl=-6;
% v_fl=KP_fl*(phi-phi_ref)+KD_fl*dphi;
% sin_psi=(v_fl-f_fl)/b_fl;
% if sin_psi < -1
%     sin_psi=-1;
% elseif sin_psi > 1
%     sin_psi=1;
% end
% 
% psi=asin(sin_psi);
% 
% dpsi=-10*(1/(m*(1.385/2)^2))*(psi0-psi);
% 
% 
% 
% beta_ref=80*pi/180;
% aux1=0.5*Ro*A*norm(va)^2;
% aux2=1/(m*r);
% e1=-va/(norm(va));
% e3=[0 0 1];
% head=dot(e1,e3);
% 
% b_alp=aux1*aux2*(-0.7*sin(psi0)*sin(beta)*sin(acos(head))-0.01*cos(beta)*head);
% f_alp=aux2*(-m*g*cos(beta)+2*m*dr*dbeta+m*r*dphi^2*cos(beta)*sin(beta)-aux1*(9.9*sin(psi0)*sin(acos(head))*sin(beta)-0.012*cos(beta)*head));
% 
% KP_alp=-9;
% KD_alp=-6;
% v_alp=KP_alp*(beta-beta_ref)+KD_alp*dbeta;
% alpha=(pi/180)*(v_alp-f_alp)/b_alp;
% 
% 
% 
% % at=0.01*(-0.7-dr);
% %     
% % end
% asd=cross(dpL,L1_G)/(norm(dpL)*norm(L1_G));
% BB=asin(asd(1))*180/pi;
if alpha>=12*pi/180
    alpha=12*pi/180;
end
if alpha<=-3*pi/180
    alpha=-3*pi/180;
end
end

== matlab function Kite/KiteSystem/XYZ ==
  data: x input; y output
function y = fcn(x)
%#codegen
 y=zeros(3,1);
% 
% R=[cos(x(2))*cos(x(3)) -sin(x(2)) -sin(x(3))*cos(x(2));
%     cos(x(3))*sin(x(2)) cos(x(2)) -sin(x(3))*sin(x(2));
%     sin(x(3)) 0 cos(x(3))];
% 
% aux=[x(1); x(2); x(3)];
% y=R*aux;


y=[x(1)*cos(x(2))*cos(x(3));
    x(1)*cos(x(3))*sin(x(2));
    x(1)*sin(x(3))];

end
